simulink model "untitled"  (R2018b)
settings: Solver=VariableStepAuto  StartTime=0.0  StopTime=3  RelTol=1e-3
libraries: dsparch4 x1, commsink2 x1, commrandsrc3 x1
settings Model: Creator=nhat  LastModifiedBy=nhat

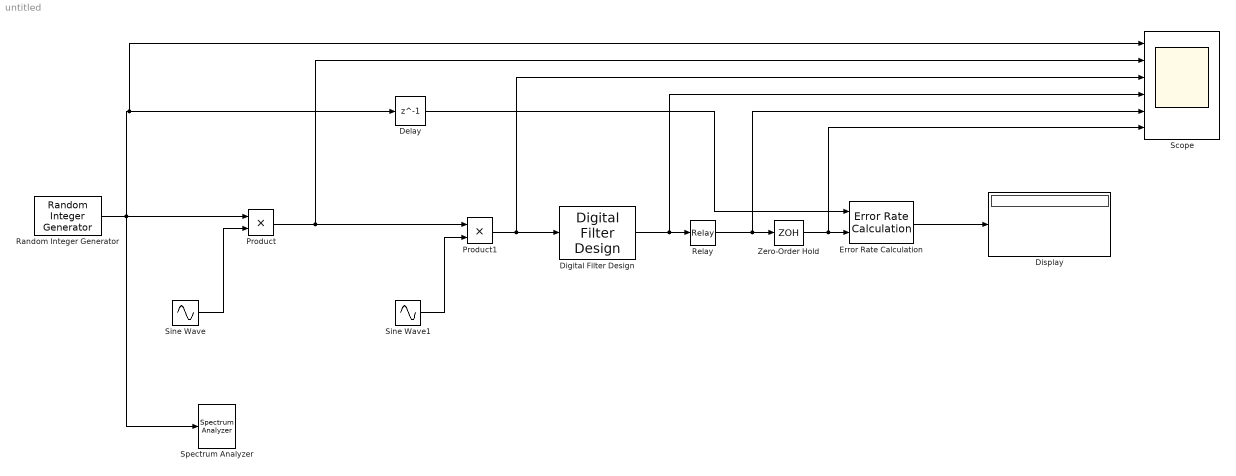
== system untitled ==
  Delay : Delay  DelayLength=1
  Digital Filter Design : dsparch4/Digital Filter Design  mwdsp_browser_bugfix_var=off
  Display : Display
  Error Rate Calculation : commsink2/Error Rate Calculation  N=0  st_delay=0  cp_mode=Entire frame  subframe=[]  PMode=Port  WsName=ErrorVec  RsMode2=off  stop=off  numErr=100  maxBits=1e6
  Product : Product
  Product1 : Product
  Random Integer Generator : commrandsrc3/Random Integer Generator  SetSize=2  SeedSource=Auto  Seed=0  SampleTime=1/1000  SamplesPerFrame=1  OutputDataType=double  SimulateUsing=Interpreted execution
  Relay : Relay  OnSwitchValue=0.3  OffSwitchValue=0.2
  Scope : Scope  NumInputPorts=6
  Sine Wave : Sin  Frequency=10000*2*pi  SampleTime=1/100000
  Sine Wave1 : Sin  Frequency=10000*pi*2  SampleTime=1/100000
  Spectrum Analyzer : SpectrumAnalyzer
  Zero-Order Hold : ZeroOrderHold  SampleTime=1/1000
  wires:
  Random Integer Generator/1 -> Spectrum Analyzer/1, Scope/1, Delay/1, Product/1
  Sine Wave/1 -> Product/2
  Product/1 -> Scope/2, Product1/1
  Sine Wave1/1 -> Product1/2
  Product1/1 -> Scope/3, Digital Filter Design/1
  Digital Filter Design/1 -> Scope/4, Relay/1
  Relay/1 -> Scope/5, Zero-Order Hold/1
  Zero-Order Hold/1 -> Scope/6, Error Rate Calculation/2
  Error Rate Calculation/1 -> Display/1
  Delay/1 -> Error Rate Calculation/1
